simulink model "hw2linearcontrolsim"  (R2025b)
settings: Solver=VariableStepAuto  StartTime=0.0  StopTime=30  RelTol=1e-3
libraries: roblocks x1
settings Model: Creator=ckitt  LastModifiedBy=Jaxba

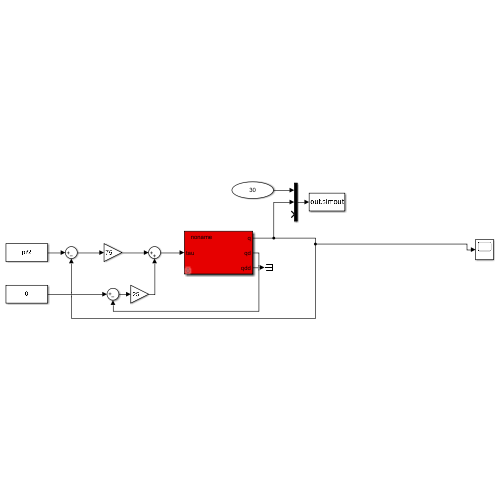
[thumbnail: Simulink's stored preview of the top-level diagram]
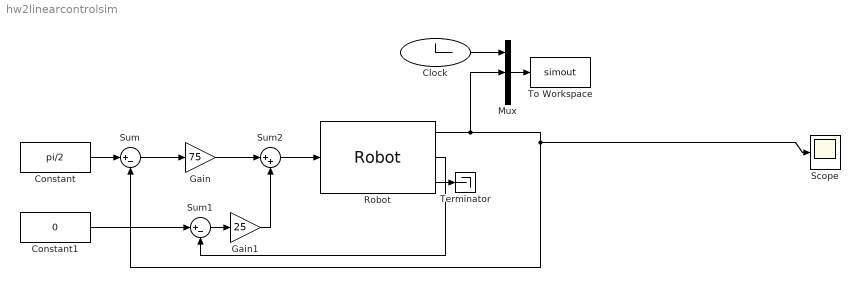
== system hw2linearcontrolsim ==
  Clock : Clock
  Constant : Constant  Value=pi/2
  Constant1 : Constant  Value=0
  Gain : Gain  Gain=75
  Gain1 : Gain  Gain=25
  Mux : Mux  Inputs=3
  Robot : roblocks/Robot  robot=SCURRbot  q0=[0 0]
  Scope : Scope
      settings: ActiveDisplayYMinimum=0.16524722890990967  ActiveDisplayYMaximum=2.4749615518328034
  Sum : Sum  Inputs=|+-
  Sum1 : Sum  Inputs=|+-
  Sum2 : Sum  Inputs=|++
  Terminator : Terminator
  To Workspace : ToWorkspace  VariableName=simout  SampleTime=-1
  wires:
  Robot/3 -> Terminator/1
  Clock/1 -> Mux/1
  Mux/1 -> To Workspace/1
  Sum/1 -> Gain/1
  Robot/1 -> Mux/2, Scope/1, Sum/2
  Constant/1 -> Sum/1
  Constant1/1 -> Sum1/1
  Robot/2 -> Sum1/2
  Gain/1 -> Sum2/1
  Sum2/1 -> Robot/1
  Sum1/1 -> Gain1/1
  Gain1/1 -> Sum2/2
